simulink model "Full_Model"  (R2024b)
settings: Solver=VariableStepAuto  StartTime=0.0  StopTime=10.0  RelTol=1e-3
libraries: shared6dof x1
settings Model: Creator=bhavy  LastModifiedBy=gtanu

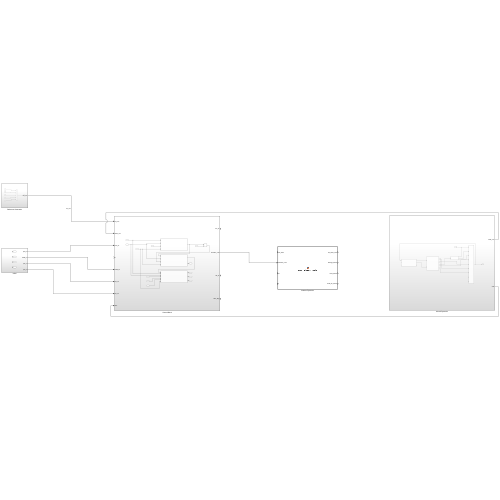
[thumbnail: Simulink's stored preview of the top-level diagram]
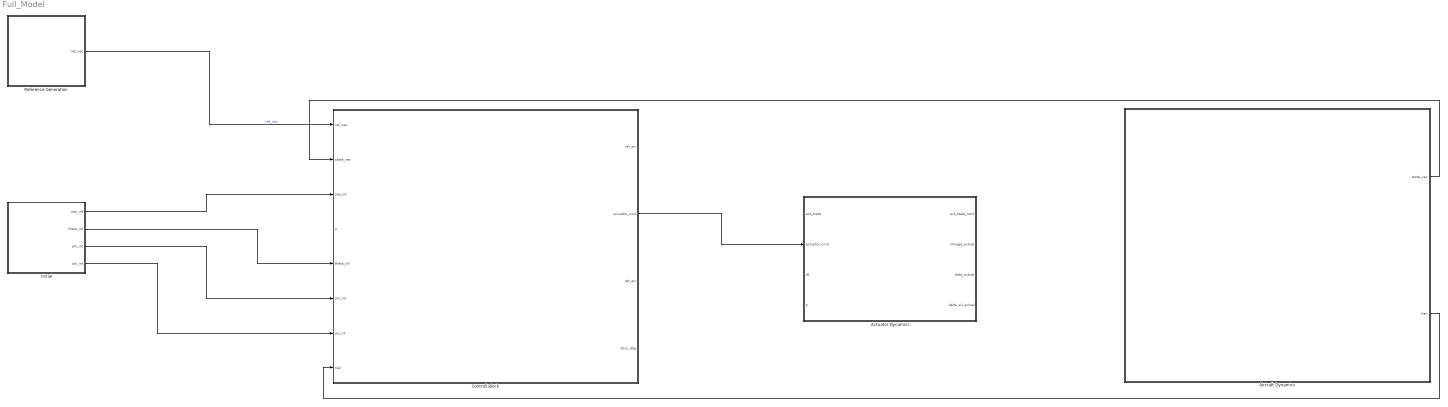
== system Full_Model ==
  Actuator Dynamics : MATLAB Function  TreatAsAtomicUnit=on
  Aircraft Dynamics : Subsystem
  Controll Block : Subsystem
  Initial : Subsystem
  Reference Generation : Subsystem
  wires:
  Reference Generation/1(ref_vec) -> Controll Block/1(ref_vec)  "ref_vec"
  Controll Block/2(actuator_cmd) -> Actuator Dynamics/2(actuator_cmd)
  Aircraft Dynamics/1(state_vec) -> Controll Block/2(state_vec)
  Aircraft Dynamics/2(Vair) -> Controll Block/8(Vair)
  Initial/1(pos_int) -> Controll Block/3(pos_int)
  Initial/2(theta_int) -> Controll Block/5(theta_int)
  Initial/3(phi_int) -> Controll Block/6(phi_int)
  Initial/4(psi_int) -> Controll Block/7(psi_int)

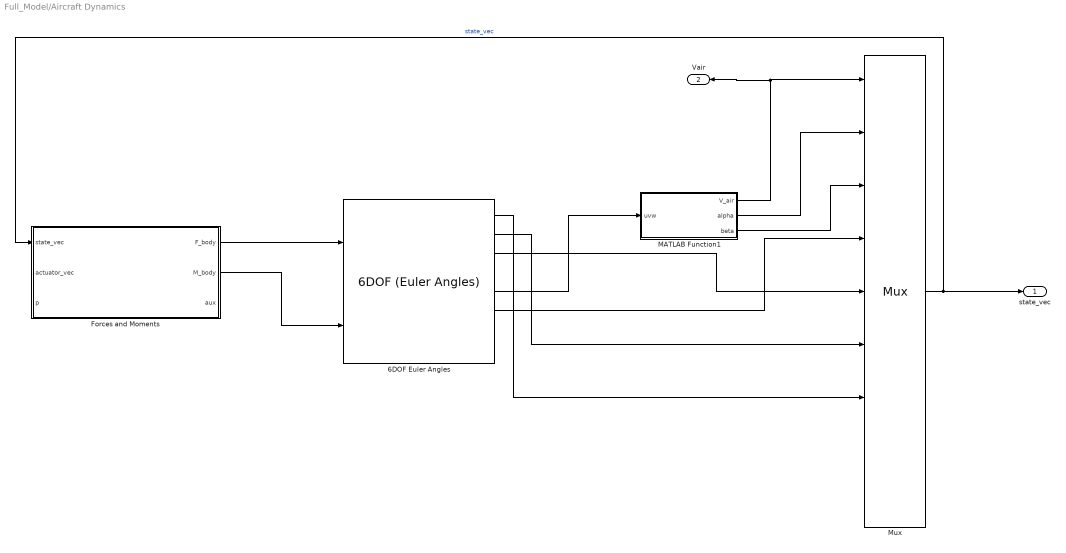
== system Full_Model/Aircraft Dynamics ==
  6DOF Euler Angles : shared6dof/6DOF (Euler Angles)  units=Metric (MKS)  mtype=Fixed  rep=Euler Angles  xme_0=[0 0 0]  Vm_0=[0 0 0]  eul_0=[0 0 0]  pm_0=[0 0 0]  mass_0=1.0  mass_e=0.5  mass_f=2.0  inertia=eye(3)  inertia_e=eye(3)  inertia_f=2*eye(3)  k_quat=1.0  vre_flag=on  abi_flag=off  aMode=0  xme_statename=''  Vm_statename=''  eul_statename=''  quat_statename=''  pm_statename=''  mass_statename=''
  Forces and Moments : MATLAB Function  TreatAsAtomicUnit=on
  MATLAB Function1 : MATLAB Function  TreatAsAtomicUnit=on
  Mux : Mux  Inputs=9
  state_vec : Outport
  Vair : Outport  Port=2
  wires:
  Forces and Moments/1(F_body) -> 6DOF Euler Angles/1
  Forces and Moments/2(M_body) -> 6DOF Euler Angles/2
  6DOF Euler Angles/5 -> MATLAB Function1/1(uvw)
  MATLAB Function1/1(V_air) -> Vair/1, Mux/1
  MATLAB Function1/2(alpha) -> Mux/2
  MATLAB Function1/3(beta) -> Mux/3
  6DOF Euler Angles/6 -> Mux/4
  6DOF Euler Angles/3 -> Mux/5
  6DOF Euler Angles/2 -> Mux/6
  6DOF Euler Angles/1 -> Mux/7
  Mux/1 -> Forces and Moments/1(state_vec), state_vec/1  "state_vec"

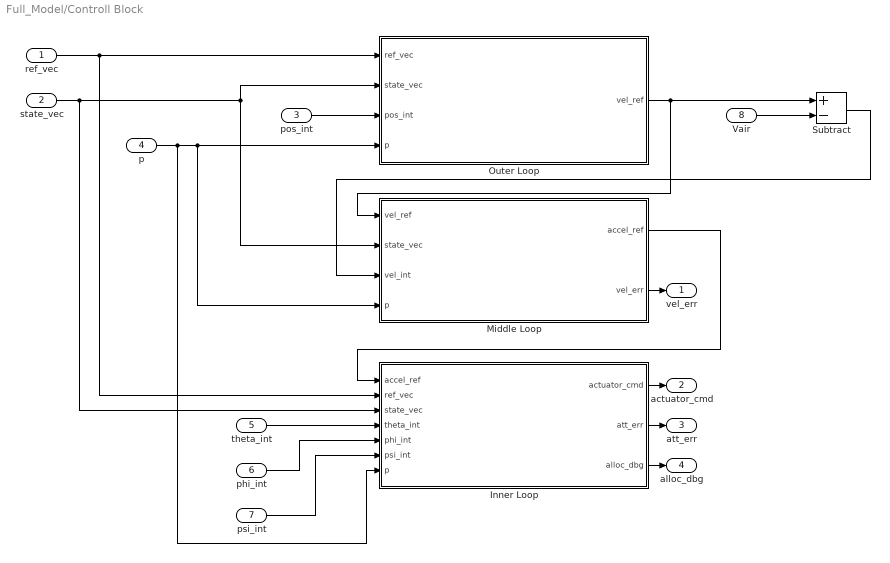
== system Full_Model/Controll Block ==
  ref_vec : Inport
  state_vec : Inport  Port=2
  pos_int : Inport  Port=3
  p : Inport  Port=4
  theta_int : Inport  Port=5
  phi_int : Inport  Port=6
  psi_int : Inport  Port=7
  Vair : Inport  Port=8
  Inner Loop : MATLAB Function  TreatAsAtomicUnit=on
  Middle Loop : MATLAB Function  TreatAsAtomicUnit=on
  Outer Loop : MATLAB Function  TreatAsAtomicUnit=on
  Subtract : Sum  Inputs=+-
  vel_err : Outport
  actuator_cmd : Outport  Port=2
  att_err : Outport  Port=3
  alloc_dbg : Outport  Port=4
  wires:
  p/1 -> Outer Loop/4(p), Middle Loop/4(p), Inner Loop/7(p)
  state_vec/1 -> Inner Loop/3(state_vec), Middle Loop/2(state_vec), Outer Loop/2(state_vec)
  Subtract/1 -> Middle Loop/3(vel_int)
  Middle Loop/2(vel_err) -> vel_err/1
  Outer Loop/1(vel_ref) -> Subtract/1, Middle Loop/1(vel_ref)
  Middle Loop/1(accel_ref) -> Inner Loop/1(accel_ref)
  ref_vec/1 -> Inner Loop/2(ref_vec), Outer Loop/1(ref_vec)
  pos_int/1 -> Outer Loop/3(pos_int)
  Inner Loop/3(alloc_dbg) -> alloc_dbg/1
  theta_int/1 -> Inner Loop/4(theta_int)
  psi_int/1 -> Inner Loop/6(psi_int)
  Inner Loop/2(att_err) -> att_err/1
  Inner Loop/1(actuator_cmd) -> actuator_cmd/1
  phi_int/1 -> Inner Loop/5(phi_int)
  Vair/1 -> Subtract/2

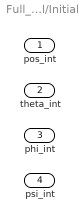
== system Full_Model/Initial ==
  pos_int : Outport
  theta_int : Outport  Port=2
  phi_int : Outport  Port=3
  psi_int : Outport  Port=4

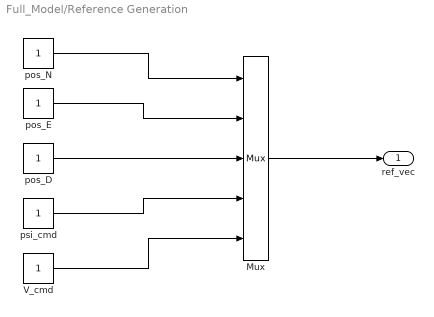
== system Full_Model/Reference Generation ==
  Mux : Mux  Inputs=5
  V_cmd : Constant
  pos_D : Constant
  pos_E : Constant
  pos_N : Constant
  psi_cmd : Constant
  ref_vec : Outport
  wires:
  pos_E/1 -> Mux/2
  V_cmd/1 -> Mux/5
  pos_D/1 -> Mux/3
  pos_N/1 -> Mux/1
  psi_cmd/1 -> Mux/4
  Mux/1 -> ref_vec/1

== matlab function Full_Model/Controll Block/Outer Loop ==
  data: ref_vec input; vel_ref output; state_vec input; pos_int input; p input
function vel_ref = dyulon_outer_loop(ref_vec, state_vec, pos_int, p) %#codegen
%DYULON_OUTER_LOOP  Position controller (outer loop).
%  Converts position error into a velocity reference command.
%  FIXED (from original): p was read via coder.extrinsic('evalin') +
%  evalin('base','p'). coder.extrinsic marks a call as MATLAB-only --
%  Embedded Coder cannot generate standalone C for it, which breaks
%  "hardware ready / code generation" for this whole function. Fixed by
%  passing p as a normal argument, matching dyulon_controller.m and
%  dyulon_actuator_dynamics.m. This requires a matching 4th inport on the
%  Simulink subsystem (see wiring notes at the end of this file / the
%  overall Simulink layout description).
%
%  INPUTS:
%    ref_vec   [5x1]  [pos_N; pos_E; pos_D; psi_cmd; V_cmd]
%    state_vec [23x1] full state vector (see dyulon_init section 19)
%    pos_int   [3x1]  integrated position error from external Discrete
%                     Integrator block (Simulink), NOT computed here.
%                     Anti-windup saturation applied at the Simulink block
%                     level using p.gains.windup_limit_outer.
%    p                parameter struct from dyulon_init.m -- FIXED: now
%                     an explicit argument, was evalin('base',...).
%
%  OUTPUTS:
%    vel_ref   [3x1]  [vN_ref; vE_ref; vD_ref]  m/s  NED frame
%
%  DESIGN NOTES:
%    - Pure PI on position. Ki starts at 0 (see dyulon_init) to avoid
%      windup during transition; raise only if steady-state position error
%      is unacceptable in simulation.
%    - Velocity commands are saturated before output. Saturation limits
%      are defined here as local constants because they are purely a
%      flight-envelope safety bound (not a tuning parameter).
%    - Integral state (pos_int) lives outside this function as a Simulink
%      Discrete Integrator block. This function only reads it.
%
%  REQUIRES (not yet in dyulon_init.m -- see accompanying integration
%  note): p.gains.outer.Kp_xy, .Ki_xy, .Kp_z, .Ki_z
%
%  STATE VECTOR INDEX REFERENCE (from dyulon_init section 19):
%    [10] pos_N  [11] pos_E  [12] pos_D
%    [13] vel_N  [14] vel_E  [15] vel_D

%% --- Unpack reference ---
pos_N_ref = ref_vec(1);
pos_E_ref = ref_vec(2);
pos_D_ref = ref_vec(3);
% ref_vec(4) = psi_cmd  - used by inner loop directly, not here
% ref_vec(5) = V_cmd    - used by inner loop directly, not here

%% --- Unpack state (position) ---
pos_N = state_vec(10);
pos_E = state_vec(11);
pos_D = state_vec(12);

%% --- Position error (NED) ---
err_N = pos_N_ref - pos_N;
err_E = pos_E_ref - pos_E;
err_D = pos_D_ref - pos_D;

%% --- PI control ---
% Integral term (pos_int) fed in from external Simulink Discrete Integrator
vN_ref = p.gains.outer.Kp_xy * err_N + p.gains.outer.Ki_xy * pos_int(1);
vE_ref = p.gains.outer.Kp_xy * err_E + p.gains.outer.Ki_xy * pos_int(2);
vD_ref = p.gains.outer.Kp_z  * err_D + p.gains.outer.Ki_z  * pos_int(3);

%% --- Output saturation ---
% Horizontal: keep well below stall (stall ~20 m/s, cap at 8 m/s for safety)
% Vertical: rate of climb target is 2 m/s from spec; cap descent at 3 m/s
vel_max_xy =  8.0;   % m/s
vel_max_dn =  3.0;   % m/s (positive = descend in NED)
vel_max_up = -2.0;   % m/s (negative = climb in NED)

vN_ref = max(min(vN_ref,  vel_max_xy), -vel_max_xy);
vE_ref = max(min(vE_ref,  vel_max_xy), -vel_max_xy);
vD_ref = max(min(vD_ref,  vel_max_dn),  vel_max_up);

vel_ref = [vN_ref; vE_ref; vD_ref];

end

== matlab function Full_Model/Aircraft Dynamics/Forces and Moments ==
  data: state_vec input; F_body output; actuator_vec input; p input; M_body output; aux output
function [F_body, M_body, aux] = dyulon_forces_moments(state_vec, actuator_vec, p)
%DYULON_FORCES_MOMENTS  Compute total forces and moments on the Dyulon airframe.
%  Rev 4 - rear motors now independently tilt (pusher convention, beta=0=down)
%  FIXED (from original): two bugs found while porting into this function:
%   (1) 'p' was used throughout but never passed in -- this function could
%       not run at all as a standalone Simulink MATLAB Function block
%       (no base-workspace evalin call either, unlike the loop functions).
%       Fixed: p is now an explicit third argument.
%   (2) actuator_vec was documented AND unpacked as 7x1 [Omega x4, beta_FL,
%       beta_FR, delta_ail] -- only front tilt. But the physics loop below
%       (`for i=1:4 ... beta_i = actuators.beta(i)`) needs beta(3) and
%       beta(4) for the rear motors, which were never assigned. Downstream,
%       dyulon_inner_loop already outputs a 9x1 actuator_cmd
%       [Omega x4, beta_FL, beta_FR, beta_RL, beta_RR, delta_ail] -- so the
%       fix is to widen this function's input to match what the rest of
%       the system already produces, not to change the inner loop.
%#codegen
% state_vec:    23x1  (see dyulon_init section 19 for index definitions)
% actuator_vec:  9x1  [Omega_FL, Omega_FR, Omega_RL, Omega_RR,
%                       beta_FL, beta_FR, beta_RL, beta_RR, delta_ail]
%
%  SIGN CONVENTION (kept as originally written, both local zeros):
%    Front motors: beta measured from straight-up    (0=up,   -90=fwd)
%    Rear  motors: beta measured from straight-down  (0=down, -90=fwd)
%    Thrust vector formula is IDENTICAL for both, because each motor's
%    beta is already expressed from its own local zero:
%      T_vec_i = T_i * [-sin(beta_i); 0; -cos(beta_i)]
%    No sign flip or per-motor conditional needed -- this was correct in
%    the original and is unchanged here.
%
%  INPUTS:
%    state_vec(23x1)     full state (dyulon_init.m Sec 19 indices)
%    actuator_vec(9x1)   [Omega_FL; Omega_FR; Omega_RL; Omega_RR;
%                          beta_FL; beta_FR; beta_RL; beta_RR; delta_ail]
%    p                   parameter struct from dyulon_init.m
%
%  OUTPUTS:
%    F_body  [3x1]  total force  in body frame  [Fx; Fy; Fz]  N
%    M_body  [3x1]  total moment in body frame  [Mx; My; Mz]  N.m
%    aux     struct of intermediate quantities for logging/debug

%% --- Unpack only what this function needs from state ---
state.V_air     = state_vec(1);
state.alpha     = state_vec(2);
state.beta_side = state_vec(3);
state.p_rate    = state_vec(4);
state.q_rate    = state_vec(5);
state.r_rate    = state_vec(6);
% [7:15] attitude and position -- not needed by forces_moments
% [16:23] actuator feedback     -- not needed by forces_moments (comes in
%                                   via actuator_vec argument instead)

%% --- Unpack actuators (FIXED: 9 elements, all 4 tilt angles present) ---
actuators.Omega(1)  = actuator_vec(1);   % Omega_FL
actuators.Omega(2)  = actuator_vec(2);   % Omega_FR
actuators.Omega(3)  = actuator_vec(3);   % Omega_RL
actuators.Omega(4)  = actuator_vec(4);   % Omega_RR
actuators.beta(1)   = actuator_vec(5);   % beta_FL
actuators.beta(2)   = actuator_vec(6);   % beta_FR
actuators.beta(3)   = actuator_vec(7);   % beta_RL  -- FIXED: was missing
actuators.beta(4)   = actuator_vec(8);   % beta_RR  -- FIXED: was missing
actuators.delta_ail = actuator_vec(9);   % index shifted 7->9

V      = state.V_air;
alpha  = state.alpha;
beta_s = state.beta_side;
p_rate = state.p_rate;
q_rate = state.q_rate;
r_rate = state.r_rate;

q_bar = 0.5 * p.rho * max(V, 0.1)^2;

%% =========================================================================
%  A. PROPELLER FORCES AND MOMENTS
%% =========================================================================
F_prop = zeros(3,1);
M_prop = zeros(3,1);
M_gyro = zeros(3,1);

V_clamped = min(V, p.prop_V_bp(end));

scale_front = interp1(p.prop_V_bp, p.KpT_front_scale, V_clamped, 'linear');
KpT_front   = p.KpT_front_0 * scale_front;
KpM_front   = p.KpM_front_0 * scale_front;

scale_rear  = interp1(p.prop_V_bp, p.KpT_rear_scale,  V_clamped, 'linear');
KpT_rear    = p.KpT_rear_0  * scale_rear;
KpM_rear    = p.KpM_rear_0  * scale_rear;

% Approximate per-rotor inertia (spinner + blades, kg.m^2)
I_rotor = 1.5e-4;
omega_body = [p_rate; q_rate; r_rate];

for i = 1:4
    Omega_i = actuators.Omega(i);

    if p.motor_type(i) == 1
        KpT_i = KpT_front;  KpM_i = KpM_front;
    else
        KpT_i = KpT_rear;   KpM_i = KpM_rear;
    end

    T_i = KpT_i * Omega_i^2;
    Q_i = KpM_i * Omega_i^2;

    % All motors have independent tilt angle from actuators.beta(i).
    % Front motors: beta measured from straight-up    (0=up,   -90=fwd)
    % Rear  motors: beta measured from straight-down  (0=down, -90=fwd)
    % Formula below is IDENTICAL for both -- convention baked into beta,
    % unchanged from the original (verified correct, kept as-is).
    beta_i = actuators.beta(i);

    T_vec = T_i * [-sin(beta_i); 0; -cos(beta_i)];

    % Reaction torque along thrust axis (opposes spin direction)
    Q_vec = -p.spin_dir(i) * Q_i * [-sin(beta_i); 0; -cos(beta_i)];

    r_i = p.r_motor(i,:)';

    F_prop = F_prop + T_vec;
    M_prop = M_prop + cross(r_i, T_vec) + Q_vec;

    % Gyroscopic coupling: H = I_rotor * Omega * spin_axis
    spin_axis = [-sin(beta_i); 0; -cos(beta_i)];
    H_rotor   = p.spin_dir(i) * I_rotor * Omega_i * spin_axis;
    M_gyro    = M_gyro + cross(omega_body, H_rotor);
end

%% =========================================================================
%  B. WING AERODYNAMICS
%% =========================================================================
if V > 2.0
    alpha_deg     = rad2deg(alpha);
    alpha_clamped = max(p.aero_alpha_deg(1), min(p.aero_alpha_deg(end), alpha_deg));

    CL = interp1(p.aero_alpha_deg, p.aero_CL, alpha_clamped, 'linear');
    CD = interp1(p.aero_alpha_deg, p.aero_CD, alpha_clamped, 'linear');
    Cm = interp1(p.aero_alpha_deg, p.aero_Cm, alpha_clamped, 'linear');

    Lift = q_bar * p.S * CL;
    Drag = q_bar * p.S * CD;

    Fx_aero =  Lift * sin(alpha) - Drag * cos(alpha);
    Fz_aero = -Lift * cos(alpha) - Drag * sin(alpha);
    Fy_aero =  q_bar * p.S * (-0.15) * beta_s;

    F_aero = [Fx_aero; Fy_aero; Fz_aero];

    Cm_total = Cm + p.Cm_q * (q_rate * p.cbar / (2 * max(V, 0.1)));
    My_aero  = q_bar * p.S * p.cbar * Cm_total;

    Cl_total = p.Cl_b  * beta_s ...
             + p.Cl_p  * (p_rate * p.b / (2 * max(V, 0.1))) ...
             + p.Cl_da * actuators.delta_ail;
    Mx_aero  = q_bar * p.S * p.b * Cl_total;

    Cn_total = p.Cn_b * beta_s + p.Cn_r * (r_rate * p.b / (2 * max(V, 0.1)));
    Mz_aero  = q_bar * p.S * p.b * Cn_total;

    M_aero = [Mx_aero; My_aero; Mz_aero];
else
    F_aero = zeros(3,1);  M_aero = zeros(3,1);
    CL = 0; CD = 0; Cm = 0; Lift = 0; Drag = 0;
end

%% =========================================================================
%  C. TOTAL FORCES AND MOMENTS
%  Gravity handled by Aerospace Blockset 6DOF (Euler Angles) block
%  internally in NED frame. Do NOT add gravity here.
%% =========================================================================
F_body = F_prop + F_aero;
M_body = M_prop + M_aero + M_gyro;

%% =========================================================================
%  D. AUX STRUCT (for Simulink logging and To Workspace blocks)
%% =========================================================================
aux.F_prop    = F_prop;
aux.F_aero    = F_aero;
aux.M_prop    = M_prop;
aux.M_aero    = M_aero;
aux.M_gyro    = M_gyro;
aux.KpT_front = KpT_front;
aux.KpT_rear  = KpT_rear;
aux.q_bar     = q_bar;
aux.CL        = CL;
aux.CD        = CD;
aux.Lift      = Lift;
aux.Drag      = Drag;

end

== matlab function Full_Model/Controll Block/Middle Loop ==
  data: vel_ref input; accel_ref output; state_vec input; vel_int input; p input; vel_err output
function [accel_ref, vel_err] = dyulon_mid_loop(vel_ref, state_vec, vel_int, p) %#codegen
%DYULON_MID_LOOP  Velocity controller (mid loop).
%  Converts velocity error into an acceleration reference command.
%  FIXED (from original): p was read via coder.extrinsic('evalin') +
%  evalin('base','p'), which blocks C code generation for this function.
%  Fixed by passing p as a normal argument (see dyulon_outer_loop_FIXED.m
%  for the same fix and the reasoning). Requires a matching 4th inport on
%  the Simulink subsystem.
%
%  INPUTS:
%    vel_ref   [3x1]  [vN_ref; vE_ref; vD_ref]   from outer loop   m/s
%    state_vec [23x1] full state vector (see dyulon_init section 19)
%    vel_int   [3x1]  integrated velocity error from external Simulink
%                     Discrete Integrator block.
%                     Anti-windup saturation: +/-p.gains.windup_limit_mid
%                     applied at the Simulink block level.
%    p                parameter struct from dyulon_init.m -- FIXED: now
%                     an explicit argument, was evalin('base',...).
%
%  OUTPUTS:
%    accel_ref [3x1]  [aN_ref; aE_ref; aD_ref]   NED frame  m/s^2
%                     These are TOTAL desired accelerations including gravity
%                     compensation - the inner loop converts to motor forces.
%    vel_err   [3x1]  current velocity error (fed to Simulink integrator
%                     input so this function and the integrator block stay
%                     in sync without recomputing the error externally)
%
%  DESIGN NOTES:
%    - NED convention: positive aD_ref = downward acceleration.
%      To hold altitude, aD_ref = 0 (gravity handled by 6DOF block).
%      To climb (pos_D decreasing = going up), aD_ref < 0.
%    - accel_ref is clamped to physically reachable values. Horizontal
%      acceleration limit chosen to keep bank angles below ~30 deg
%      (tan(30) * g ~= 5.7 m/s^2). Vertical limit from T/W ratio.
%    - This function only outputs the proportional + integral correction.
%      The inner loop handles gravity compensation internally via the
%      collective thrust term.
%
%  REQUIRES (not yet in dyulon_init.m -- see accompanying integration
%  note): p.gains.mid.Kp_xy, .Ki_xy, .Kp_z, .Ki_z
%
%  STATE VECTOR INDEX REFERENCE:
%    [13] vel_N  [14] vel_E  [15] vel_D  m/s NED

%% --- Unpack velocity from state ---
vel_N = state_vec(13);
vel_E = state_vec(14);
vel_D = state_vec(15);

%% --- Velocity error ---
err_N = vel_ref(1) - vel_N;
err_E = vel_ref(2) - vel_E;
err_D = vel_ref(3) - vel_D;

vel_err = [err_N; err_E; err_D];

%% --- PI acceleration command ---
aN_ref = p.gains.mid.Kp_xy * err_N + p.gains.mid.Ki_xy * vel_int(1);
aE_ref = p.gains.mid.Kp_xy * err_E + p.gains.mid.Ki_xy * vel_int(2);
aD_ref = p.gains.mid.Kp_z  * err_D + p.gains.mid.Ki_z  * vel_int(3);

%% --- Output saturation ---
% Horizontal: bank angle limited to ~30 deg implicitly (5.7 m/s^2)
% Vertical: T/W = 1.4 gives max upward accel of 0.4*g ~= 3.9 m/s^2 net of gravity
accel_max_xy  =  5.7;          % m/s^2
accel_max_dn  =  0.4 * p.g;    % m/s^2  (positive = push downward in NED, rare)
accel_max_up  = -0.4 * p.g;    % m/s^2  (negative = push upward in NED, climb)

aN_ref = max(min(aN_ref,  accel_max_xy), -accel_max_xy);
aE_ref = max(min(aE_ref,  accel_max_xy), -accel_max_xy);
aD_ref = max(min(aD_ref,  accel_max_dn),  accel_max_up);

accel_ref = [aN_ref; aE_ref; aD_ref];

end

== matlab function Full_Model/Controll Block/Inner Loop ==
  data: accel_ref input; actuator_cmd output; ref_vec input; state_vec input; theta_int input; phi_int input; psi_int input; p input; att_err output; alloc_dbg output
function [actuator_cmd, att_err, alloc_dbg] = dyulon_inner_loop(...
    accel_ref, ref_vec, state_vec, theta_int, phi_int, psi_int, p) %#codegen
%DYULON_INNER_LOOP  Attitude + control allocation (inner loop).
%
%  Takes desired acceleration from the mid loop and the full state, and
%  outputs motor speed (Omega) and tilt angle (beta) commands for all 4
%  motors plus aileron deflection.
%
%  The function is structured in five sequential stages:
%    1. Unpack state and compute blend factor
%    2. Compute attitude reference (theta_ref, phi_ref, psi_ref)
%    3. AoA protection - saturate theta_ref if stall risk detected,
%       flag that motor speed compensation is needed
%    4. PID attitude control -> desired angular accelerations
%    5. Control allocation:
%         a. Compute collective thrust needed (vertical + forward)
%         b. Distribute among motors using 2-DOF per motor (Omega + beta)
%            DOF weighting from p.alloc_weights (currently 50/50)
%            Tilt perturbation bounded by stage-dependent limits from
%            p.tilt_limits, interpolated continuously via blend
%         c. Apply motor speed compensation if AoA was saturated
%         d. Saturate all outputs against hard mechanical/electrical limits
%
%  INPUTS:
%    accel_ref  [3x1]  [aN; aE; aD]  NED  m/s²   from mid loop
%    ref_vec    [5x1]  [pos_N; pos_E; pos_D; psi_cmd; V_cmd]
%    state_vec  [23x1] full state (see dyulon_init section 19)
%    theta_int  [1x1]  integrated pitch error  (external Discrete Integrator)
%    phi_int    [1x1]  integrated roll error   (external Discrete Integrator)
%    psi_int    [1x1]  integrated yaw error    (external Discrete Integrator)
%
%  OUTPUTS:
%    actuator_cmd [9x1]  [Omega_FL; Omega_FR; Omega_RL; Omega_RR;
%                          beta_FL;  beta_FR;  beta_RL;  beta_RR;
%                          delta_ail]
%    att_err      [3x1]  [theta_err; phi_err; psi_err]  for integrator input
%    alloc_dbg    [6x1]  debug: [blend; theta_ref; phi_ref;
%                                aoa_saturated; Fz_motors; Fx_motors]
%
%  STATE VECTOR INDEX REFERENCE (dyulon_init section 19):
%    [1]  V_air   [2]  alpha   [3]  beta_side
%    [4]  p_rate  [5]  q_rate  [6]  r_rate
%    [7]  phi     [8]  theta   [9]  psi
%    [10:12] pos  [13:15] vel
%    [16] beta_FL [17] beta_FR [18] beta_RL [19] beta_RR
%    [20] Omega_FL [21] Omega_FR [22] Omega_RL [23] Omega_RR
%
%  FIXED (from original): p was read via coder.extrinsic('evalin') +
%  evalin('base','p'), which blocks Embedded Coder C generation for this
%  function -- same issue and same fix as dyulon_outer_loop / dyulon_mid_loop.
%  p is now the 7th argument. Requires a matching 7th inport on the
%  Simulink subsystem.

%% =========================================================================
%  STAGE 1 - UNPACK STATE
%% =========================================================================
V_air   = state_vec(1);
alpha   = state_vec(2);   % rad, angle of attack
p_rate  = state_vec(4);   % rad/s, roll rate
q_rate  = state_vec(5);   % rad/s, pitch rate
r_rate  = state_vec(6);   % rad/s, yaw rate
phi     = state_vec(7);   % rad, roll angle
theta   = state_vec(8);   % rad, pitch angle
psi     = state_vec(9);   % rad, yaw angle

% Current actual tilt and speed (feedback from actuator model output)
beta_actual  = state_vec(16:19);   % [FL; FR; RL; RR] rad
% Omega_actual = state_vec(20:23); % available if needed for feedforward

psi_cmd = ref_vec(4);

%% =========================================================================
%  STAGE 2 - BLEND FACTOR (single source of truth, same formula as doc)
%% =========================================================================
blend = max(0.0, min(1.0, (V_air - p.V_blend_lo) / (p.V_blend_hi - p.V_blend_lo)));

%% =========================================================================
%  STAGE 3 - ATTITUDE REFERENCE
%
%  theta_ref: interpolate between hover (0 rad) and cruise (alpha_bestLD)
%  phi_ref:   derived from lateral acceleration demand (coordinated turn)
%  psi_ref:   commanded heading from ref_vec
%
%  NOTE: accel_ref is in NED. To get body-frame lateral accel demand
%  (used for bank angle reference), we rotate using current heading psi.
%% =========================================================================

% Pitch reference - blend from hover to best-L/D AoA in cruise
theta_hover  = 0.0;
theta_cruise = deg2rad(p.alpha_bestLD_deg);   % trim at best L/D
theta_ref    = (1.0 - blend) * theta_hover + blend * theta_cruise;

% Roll reference from lateral acceleration demand (NED -> body lateral)
% Body-frame lateral accel ≈ -sin(psi)*aN + cos(psi)*aE  for small phi
ay_body  = -sin(psi) * accel_ref(1) + cos(psi) * accel_ref(2);
phi_ref  = atan2(ay_body, p.g);   % coordinated turn bank angle
phi_ref  = max(min(phi_ref, deg2rad(30)), deg2rad(-30));  % limit bank to ±30 deg

psi_ref  = psi_cmd;

%% =========================================================================
%  STAGE 4 - AoA PROTECTION
%
%  If current alpha approaches stall, override theta_ref with the
%  protection ceiling and flag that extra motor speed is needed to meet
%  the original lift demand. The motor compensation is applied in Stage 6.
%
%  Protection band from dyulon_init:
%    p.alpha_protect_lo_deg  - lower bound (avoid negative stall)
%    p.alpha_protect_hi_deg  - upper bound (stall margin = stall_AoA - 2 deg)
%% =========================================================================
alpha_deg       = rad2deg(alpha);
aoa_saturated   = 0.0;   % flag: 0 = normal, 1 = upper, -1 = lower

if alpha_deg >= p.alpha_protect_hi_deg
    % Approaching stall - cap theta_ref so AoA stops increasing
    % We cannot pitch further nose-up, but we CAN increase motor speed
    theta_ref     = deg2rad(p.alpha_protect_hi_deg);
    aoa_saturated = 1.0;
elseif alpha_deg <= p.alpha_protect_lo_deg
    % Approaching negative stall (e.g. aggressive pushover)
    theta_ref     = deg2rad(p.alpha_protect_lo_deg);
    aoa_saturated = -1.0;
end

%% =========================================================================
%  STAGE 5 - PID ATTITUDE CONTROL
%
%  Uses direct rate feedback for derivative term (not d(error)/dt) to
%  avoid differentiating noisy angle measurements. This structure is
%  directly portable to ArduPilot's rate-feedback PID architecture.
%
%    pitch output = Kp*(theta_ref-theta) + Ki*theta_int - Kd*q_rate
%    roll  output = Kp*(phi_ref-phi)     + Ki*phi_int   - Kd*p_rate
%    yaw   output = Kp*(psi_ref-psi)     + Ki*psi_int   - Kd*r_rate
%
%  Output is a desired angular acceleration [rad/s²] for pitch and roll,
%  and a desired yaw rate correction [rad/s] for yaw (Kd_psi = 0 default).
%  These drive the force allocation in Stage 6.
%% =========================================================================

% Attitude errors (fed back out as att_err for Simulink integrator inputs)
theta_err = theta_ref - theta;
phi_err   = phi_ref   - phi;
psi_err   = psi_ref   - psi;

% Wrap yaw error to [-pi, pi]
psi_err = mod(psi_err + pi, 2*pi) - pi;

att_err = [theta_err; phi_err; psi_err];

% PID outputs (desired angular accelerations / rate corrections)
pitch_cmd = p.gains.inner.Kp_theta * theta_err ...
          + p.gains.inner.Ki_theta  * theta_int ...
          - p.gains.inner.Kd_theta  * q_rate;

roll_cmd  = p.gains.inner.Kp_phi   * phi_err ...
          + p.gains.inner.Ki_phi    * phi_int ...
          - p.gains.inner.Kd_phi    * p_rate;

yaw_cmd   = p.gains.inner.Kp_psi   * psi_err ...
          + p.gains.inner.Ki_psi    * psi_int ...
          - p.gains.inner.Kd_psi    * r_rate;

% Convert angular acceleration demands to differential force demands
% pitch_force = Iyy * pitch_cmd / moment_arm (front-rear x distance)
x_arm   = p.x_front - p.x_rear;   % m  total front-to-rear moment arm
y_arm_f = abs(p.r_motor(1,2));     % m  front lateral arm (roll)
y_arm_r = abs(p.r_motor(3,2));     % m  rear  lateral arm (roll)
y_arm   = 0.5 * (y_arm_f + y_arm_r);  % average for roll allocation

delta_F_pitch = p.Iyy * pitch_cmd / x_arm;   % N  differential vertical force front vs rear
delta_F_roll  = p.Ixx * roll_cmd  / y_arm;   % N  differential vertical force left vs right
delta_F_yaw   = p.Izz * yaw_cmd;             % N·m  yaw torque demand (met by reaction torques)

%% =========================================================================
%  STAGE 6 - COLLECTIVE THRUST DEMAND
%
%  Vertical force needed from motors:
%    In hover:  motors provide all lift = mass * (g + az_cmd)
%    In cruise: wing provides blend fraction of lift, motors provide rest
%
%  Forward force needed from motors:
%    In hover:  from aN/aE demands (small, met by tilt)
%    In cruise: from drag balance (met primarily by rear motors)
%
%  accel_ref is NED (positive D = downward). To get vertical demand in
%  body frame (z-down), Fz_needed is the upward force = mass*(g - aD_NED)
%  because aD_NED > 0 means accelerating downward (reducing lift demand).
%
%  Wing lift available at current alpha and airspeed:
%    Lift_avail = 0.5*rho*V^2*S*CL(alpha) - looked up from LUT
%  Motor vertical demand = total_needed - blend*Lift_avail
%% =========================================================================

% Total upward force needed [body frame, positive = up, so subtract aD]
Fz_total_needed = p.mass * (p.g - accel_ref(3));   % accel_ref(3) = aD_NED

% Wing lift available now (interpolate from LUT at current alpha)
alpha_deg_clamped = max(p.aero_alpha_deg(1), min(p.aero_alpha_deg(end), alpha_deg));
CL_now     = interp1(p.aero_alpha_deg, p.aero_CL, alpha_deg_clamped, 'linear');
Lift_avail = 0.5 * p.rho * max(V_air, 0.1)^2 * p.S * CL_now;

% Motor vertical demand (wing takes blend fraction, motors take the rest)
Fz_motors = Fz_total_needed - blend * Lift_avail;
Fz_motors = max(Fz_motors, 0.0);   % motors cannot pull downward

% Forward force demand (body x-axis)
% In NED: ax_body ≈ cos(psi)*aN + sin(psi)*aE  for small phi/theta
ax_body   = cos(psi) * accel_ref(1) + sin(psi) * accel_ref(2);
% Drag at current condition (for feedforward in cruise)
CD_now    = interp1(p.aero_alpha_deg, p.aero_CD, alpha_deg_clamped, 'linear');
Drag_now  = 0.5 * p.rho * max(V_air, 0.1)^2 * p.S * CD_now;
Fx_motors = p.mass * ax_body + Drag_now;   % overcome drag + accelerate forward

% Front/rear collective split (from frac_front / frac_rear)
Fz_front = p.frac_front * Fz_motors;
Fz_rear  = p.frac_rear  * Fz_motors;
Fx_front = p.frac_front * Fx_motors;
Fx_rear  = p.frac_rear  * Fx_motors;

%% =========================================================================
%  STAGE 7 - 2-DOF CONTROL ALLOCATION PER MOTOR GROUP
%
%  Each motor has two DOFs: Omega (speed -> thrust magnitude) and beta
%  (tilt -> thrust direction). For a given thrust VECTOR demand [Fx; Fz],
%  there are infinitely many (Omega, beta) combinations that satisfy it.
%  The allocation weight (p.alloc_weights) splits the correction between
%  the two DOFs: at 0.5/0.5, half the correction is attempted via beta
%  change and half via Omega change.
%
%  PRIMARY tilt target (blend-driven, stage-level command):
%    Front: beta_front_primary = beta_front_rest + (-pi/2 - beta_front_rest)*blend
%           = 0 + (-90 - 0)*blend = -90*blend deg
%           (0 deg in hover = straight up, -90 deg in cruise = forward)
%
%    Rear:  beta_rear_primary  = beta_rear_rest + (-pi/2 - beta_rear_rest)*blend
%           = -20 + (-90 - (-20))*blend = -20 - 70*blend  [deg]
%           At blend=0 (hover):      beta = -20 deg  (94% up, 34% fwd)
%           At blend=0.5 (transit):  beta = -55 deg  (82% fwd, 57% up)
%           At blend=1 (cruise):     beta = -90 deg  (100% fwd, 0% up)
%           The -100 deg hard stop gives ±10 deg perturbation room in cruise.
%
%  PERTURBATION on top of primary (for attitude correction via tilt):
%    Interpolated from p.tilt_limits vs blend continuously.
%    Front perturb: 2 deg (hover) -> 10 deg (cruise)
%    Rear  perturb: 8 deg (hover) ->  2 deg (cruise)
%
%  MOTOR SPEED from the remaining force demand not met by tilt change.
%
%  All outputs clamped to hard limits from p before exit.
%% =========================================================================

% --- Tilt perturbation limits at current blend (continuous interp) ---
front_perturb_rad = interp1(p.tilt_limits.V_bp, ...
                            p.tilt_limits.front_perturb_rad_bp, ...
                            V_air, 'linear', 'extrap');
front_perturb_rad = max(0, min(front_perturb_rad, deg2rad(15)));

rear_perturb_rad  = interp1(p.tilt_limits.V_bp, ...
                             p.tilt_limits.rear_perturb_rad_bp, ...
                             V_air, 'linear', 'extrap');
rear_perturb_rad  = max(0, min(rear_perturb_rad, deg2rad(15)));

% --- Primary tilt commands (stage-level blend schedule) ---
% Front: 0 (hover) -> -pi/2 (cruise), referenced from front zero (up)
beta_front_primary = p.beta_front_rest + (-pi/2 - p.beta_front_rest) * blend;

% Rear: -100deg (hover) -> -90deg (cruise), referenced from rear zero (down)
beta_rear_primary  = p.beta_rear_rest  + (-pi/2 - p.beta_rear_rest)  * blend;

% --- Attitude correction via tilt (pitch) ---
% Positive pitch_correction: want more nose-up = front motors tilt back
% (less forward component = increase beta toward 0) or rear motors
% tilt more forward (decrease beta, more negative for rear convention).
% Scale delta_F_pitch to a tilt perturbation angle via a linearisation:
% dFz/dbeta ≈ -T_front * cos(beta_primary) at operating point
% Use a soft gain rather than exact inversion (plant uncertainty too high
% for exact inversion at this stage)
pitch_tilt_gain_front = 0.003;  % rad/N  - tune in sim
pitch_tilt_gain_rear  = 0.003;  % rad/N

delta_beta_pitch_front = p.alloc_weights.tilt_share * pitch_tilt_gain_front * delta_F_pitch;
delta_beta_pitch_rear  = p.alloc_weights.tilt_share * pitch_tilt_gain_rear  * (-delta_F_pitch);

% Clamp tilt perturbation to stage-dependent limit
delta_beta_pitch_front = max(min(delta_beta_pitch_front,  front_perturb_rad), -front_perturb_rad);
delta_beta_pitch_rear  = max(min(delta_beta_pitch_rear,   rear_perturb_rad),  -rear_perturb_rad);

% --- Roll correction: only via motor SPEED (L/R differential Omega) ---
% Tilt does not help with roll (both L and R motors on same fore-aft axis).
% Roll entirely via Omega differential, ignoring alloc_weights for roll axis.
% (alloc_weights applies only to pitch/thrust axes where tilt can help)

% --- Compute required thrust magnitudes per motor ---
% Remaining vertical force after tilt perturbation (Omega carries the rest)
% Front motors: each provides Fz_front/2 ± roll differential
KpT_front_now = p.KpT_front_0 * interp1(p.prop_V_bp, p.KpT_front_scale, ...
                min(V_air, p.prop_V_bp(end)), 'linear');
KpT_rear_now  = p.KpT_rear_0  * interp1(p.prop_V_bp, p.KpT_rear_scale, ...
                min(V_air, p.prop_V_bp(end)), 'linear');

% Collective Omega from vertical + forward demand
% |T_front| = sqrt(Fz_front^2 + Fx_front^2) per motor (vector magnitude)
T_front_mag = sqrt((Fz_front/2)^2 + (Fx_front/2)^2);
T_rear_mag  = sqrt((Fz_rear/2)^2  + (Fx_rear/2)^2);

% Omega_collective = sqrt(T_mag / KpT)  only for the Omega share
T_front_omega_share = T_front_mag * p.alloc_weights.omega_share;
T_rear_omega_share  = T_rear_mag  * p.alloc_weights.omega_share;

% Add back the tilt share (tilt handles the rest; Omega only sees its share)
% In practice the full T is still needed, but the tilt adjusts direction
% so the effective Omega demand is based on vector magnitude not just vertical
Omega_front_col = sqrt(max(T_front_mag / max(KpT_front_now, 1e-9), 0));
Omega_rear_col  = sqrt(max(T_rear_mag  / max(KpT_rear_now,  1e-9), 0));

% --- Signed-sqrt for attitude differential Omega corrections ---
% Uses sign(x)*sqrt(|x|) to allow bidirectional corrections without
% clipping negative demands to zero (Rev 3 bugfix carried forward).
signed_sqrt = @(x) sign(x) * sqrt(abs(x));

% Pitch correction via motor speed (Omega share of delta_F_pitch)
dF_pitch_omega_front = p.alloc_weights.omega_share * ( delta_F_pitch / 2);
dF_pitch_omega_rear  = p.alloc_weights.omega_share * (-delta_F_pitch / 2);
dOmega_pitch_front   = signed_sqrt(dF_pitch_omega_front / max(KpT_front_now, 1e-9));
dOmega_pitch_rear    = signed_sqrt(dF_pitch_omega_rear  / max(KpT_rear_now,  1e-9));

% Roll correction fully via motor speed differential
dF_roll  = delta_F_roll / 2;   % per motor, symmetric
dOmega_roll_f = signed_sqrt(dF_roll / max(KpT_front_now, 1e-9));
dOmega_roll_r = signed_sqrt(dF_roll / max(KpT_rear_now,  1e-9));

% --- Yaw correction via differential reaction torque ---
% Yaw authority is weak (no fin). Differential Omega changes reaction torque.
% KpM/KpT ratio gives torque per unit thrust, so:
% delta_Q_yaw must equal delta_F_yaw
% delta_Q = KpM * delta_Omega^2 (approximately: 2*KpM*Omega*dOmega for small dOmega)
% Use simple proportional split: increase CCW pair, decrease CW pair
% Spin dirs: FL=-1(CCW), FR=+1(CW), RL=+1(CW), RR=-1(CCW)
KpM_front_now = p.KpM_front_0 * interp1(p.prop_V_bp, p.KpM_front_scale, ...
                min(V_air, p.prop_V_bp(end)), 'linear');
yaw_gain = 0.001;  % rad/s per N·m yaw demand - soft gain, tune in sim
dOmega_yaw = yaw_gain * yaw_cmd;  % same magnitude, sign varies by spin direction below

% --- Final per-motor tilt angles ---
beta_FL = beta_front_primary + delta_beta_pitch_front;
beta_FR = beta_front_primary + delta_beta_pitch_front;  % same pitch correction
beta_RL = beta_rear_primary  + delta_beta_pitch_rear;
beta_RR = beta_rear_primary  + delta_beta_pitch_rear;

% Hard clamp to mechanical stops (from p.beta_motor_min / max)
beta_FL = max(min(beta_FL, p.beta_motor_max(1)), p.beta_motor_min(1));
beta_FR = max(min(beta_FR, p.beta_motor_max(2)), p.beta_motor_min(2));
beta_RL = max(min(beta_RL, p.beta_motor_max(3)), p.beta_motor_min(3));
beta_RR = max(min(beta_RR, p.beta_motor_max(4)), p.beta_motor_min(4));

% --- Final per-motor Omega ---
% Spin dirs: FL=-1, FR=+1, RL=+1, RR=-1
% Roll: right motors (FR, RR) go up = increase Omega_R to roll left
%   -> FL decreases, FR increases, RL decreases, RR increases (or signs flip)
%   Convention: positive roll_cmd = roll right = right wing goes down
%               = left motors increase, right motors decrease
Omega_FL = Omega_front_col + dOmega_pitch_front - dOmega_roll_f - p.spin_dir(1)*dOmega_yaw;
Omega_FR = Omega_front_col + dOmega_pitch_front + dOmega_roll_f - p.spin_dir(2)*dOmega_yaw;
Omega_RL = Omega_rear_col  + dOmega_pitch_rear  - dOmega_roll_r - p.spin_dir(3)*dOmega_yaw;
Omega_RR = Omega_rear_col  + dOmega_pitch_rear  + dOmega_roll_r - p.spin_dir(4)*dOmega_yaw;

%% =========================================================================
%  STAGE 8 - AoA SATURATION MOTOR SPEED COMPENSATION
%
%  If AoA was saturated (aoa_saturated != 0), the original lift demand
%  cannot be met by pitching further. Instead, distribute the unmet lift
%  demand as additional collective motor speed across all 4 motors, split
%  proportionally by p.alloc_weights.omega_share vs wing contribution.
%
%  Weight: 50% front, 50% rear (p.alloc_weights is 50/50 globally).
%% =========================================================================
if abs(aoa_saturated) > 0.5
    % Estimate unmet lift: how much MORE vertical force is needed above
    % what the current theta_ref + current alpha provides?
    % Approximation: unmet = original Fz_total_needed - current Lift_avail - Fz_motors
    % In practice the integrators will handle slow residual; this compensation
    % is for fast transient saturation events only.
    Lift_at_protected_aoa = 0.5 * p.rho * max(V_air,0.1)^2 * p.S * CL_now;
    Fz_unmet = max(Fz_total_needed - Lift_at_protected_aoa - Fz_motors, 0);

    % Split unmet force across all 4 motors proportionally
    dF_comp_front = Fz_unmet * p.alloc_weights.omega_share * p.frac_front / 2;
    dF_comp_rear  = Fz_unmet * p.alloc_weights.omega_share * p.frac_rear  / 2;

    dOmega_comp_front = signed_sqrt(dF_comp_front / max(KpT_front_now, 1e-9));
    dOmega_comp_rear  = signed_sqrt(dF_comp_rear  / max(KpT_rear_now,  1e-9));

    Omega_FL = Omega_FL + dOmega_comp_front;
    Omega_FR = Omega_FR + dOmega_comp_front;
    Omega_RL = Omega_RL + dOmega_comp_rear;
    Omega_RR = Omega_RR + dOmega_comp_rear;
end

%% =========================================================================
%  STAGE 9 - AILERON (blend-weighted, suppressed in hover)
%
%  In hover (blend=0): ailerons too slow to be effective, command = 0.
%  In cruise (blend=1): ailerons are primary roll actuator.
%  roll_cmd is in rad/s² (desired roll acceleration). Scale to aileron
%  deflection via static effectiveness (p.Cl_da, wing geometry).
%  Aileron effectiveness: M_roll = q_bar * S * b * Cl_da * delta_ail
%    -> delta_ail = Ixx * roll_cmd / (q_bar * S * b * Cl_da)
%  Suppressed in low-q (slow flight) by blend weight.
%% =========================================================================
q_bar_now   = 0.5 * p.rho * max(V_air, 0.1)^2;
ail_denom   = q_bar_now * p.S * p.b * p.Cl_da;
if abs(ail_denom) > 1e-6
    delta_ail_raw = blend * (p.Ixx * roll_cmd / ail_denom);
else
    delta_ail_raw = 0;
end
delta_ail = max(min(delta_ail_raw, p.aileron_max), p.aileron_min);

%% =========================================================================
%  STAGE 10 - FINAL SATURATION OF MOTOR SPEEDS
%% =========================================================================
Omega_FL = max(min(Omega_FL, p.Omega_max(1)), p.Omega_min(1));
Omega_FR = max(min(Omega_FR, p.Omega_max(2)), p.Omega_min(2));
Omega_RL = max(min(Omega_RL, p.Omega_max(3)), p.Omega_min(3));
Omega_RR = max(min(Omega_RR, p.Omega_max(4)), p.Omega_min(4));

%% =========================================================================
%  OUTPUTS
%% =========================================================================
actuator_cmd = [Omega_FL; Omega_FR; Omega_RL; Omega_RR;
                beta_FL;  beta_FR;  beta_RL;  beta_RR;
                delta_ail];

% Debug vector for Simulink logging (To Workspace block)
alloc_dbg = [blend; theta_ref; phi_ref; aoa_saturated; Fz_motors; Fx_motors];

== matlab function Full_Model/Actuator Dynamics ==
  data: act_state input; act_state_next output; actuator_cmd input; dt input; p input; Omega_actual output; beta_actual output; delta_ail_actual output
function [act_state_next, Omega_actual, beta_actual, delta_ail_actual] = ...
    dyulon_actuator_dynamics(act_state, actuator_cmd, dt, p) %#codegen
%DYULON_ACTUATOR_DYNAMICS  Discrete-time actuator lag/rate-limit/saturation.
%  Models the REAL hardware: 4x ESC+motor (speed loop), 4x direct-drive
%  gearmotor tilt actuator (NOT a servo), and the aileron servo.
%
%  COMPATIBILITY CHANGE (this revision): earlier version assumed a single
%  unified beta convention (0=horizontal, pi/2=vertical, shared front/rear
%  limits). The controller cascade (dyulon_inner_loop etc.) instead uses
%  TWO local zeros -- front: 0=up,-90deg=fwd; rear: 0=down,-90deg=fwd --
%  per motor, with PER-MOTOR limits (p.beta_motor_min/max, 4x1 each),
%  not shared front/rear bounds. This function's 2nd-order tilt dynamics
%  are convention-agnostic (they only act on the numeric difference
%  beta_cmd - beta, regardless of what zero means physically), so ONLY
%  the saturation limits changed -- from p.beta_min_front/rear (2 shared
%  values) to p.beta_motor_min/max (4x1, one per motor). No other logic
%  needed to change.
%
%  INPUT SHAPE CHANGE: now takes the actual 9x1 actuator_cmd vector
%  dyulon_inner_loop already produces
%  ([Omega_FL;Omega_FR;Omega_RL;Omega_RR; beta_FL;beta_FR;beta_RL;beta_RR;
%  delta_ail]) directly, instead of two separate 4x1 arguments -- avoids
%  an extra Demux/Selector in Simulink between inner_loop and this block.
%  Aileron is modelled here too now (1st-order lag + saturation), since it
%  is part of the same actuator_cmd vector and was previously handled
%  nowhere in the actuator-dynamics stage.
%
%  HARDWARE-READY BY DESIGN:
%    No persistent/global state and no Simulink-specific constructs. All
%    state is explicit in (act_state) and out (act_state_next); the only
%    external input is dt (seconds) and the parameter struct p. Same
%    signature a PX4 module would use per control-loop tick:
%    state_next = f(state, cmd, dt, params).
%
%    INTERNAL SUB-STEPPING: forward-Euler integration of the tilt 2nd-order
%    dynamics requires dt < p.dt_actuator_max (~0.1/tilt_omega_n) for
%    numerical stability. If the caller's dt exceeds this, this function
%    automatically sub-steps internally at p.dt_actuator_max so the OUTER
%    control loop rate is decoupled from the actuator model's numerical
%    stability requirement -- call this once per controller tick
%    regardless of dt; it self-subdivides. Port the same sub-stepping
%    logic to firmware if the flight computer's actuator-update rate is
%    slower than this bound.
%
%  ACTUATOR STATE LAYOUT (act_state, struct):
%    act_state.Omega(4)      rad/s   current motor speed (1st-order lag state)
%    act_state.beta(4)       rad     current tilt angle   (2nd-order lag state 1)
%    act_state.beta_dot(4)   rad/s   current tilt rate    (2nd-order lag state 2)
%    act_state.delta_ail     rad     current aileron deflection (1st-order lag)
%
%  INPUTS:
%    actuator_cmd(9x1)  [Omega_FL; Omega_FR; Omega_RL; Omega_RR;
%                         beta_FL;  beta_FR;  beta_RL;  beta_RR;
%                         delta_ail]   commanded values from dyulon_inner_loop,
%                         PRE-actuator-dynamics (this function's whole job
%                         is to turn these into what the hardware actually
%                         does a moment later)
%    dt                 s    CALLER's control step (any value -- this
%                              function sub-steps internally as needed)
%    p                       parameter struct from dyulon_init.m
%
%  OUTPUTS:
%    act_state_next            updated actuator state for next call
%    Omega_actual(4x1)  rad/s  actual (lagged, saturated) motor speed
%    beta_actual(4x1)   rad    actual (lagged, rate-limited, saturated) tilt
%    delta_ail_actual   rad    actual (lagged, saturated) aileron deflection
%    All three "actual" outputs feed dyulon_forces_moments as the 9x1
%    actuator_vec: [Omega_actual; beta_actual; delta_ail_actual].

%% --- Unpack the flat command vector ---
Omega_cmd = actuator_cmd(1:4);
beta_cmd  = actuator_cmd(5:8);
delta_ail_cmd = actuator_cmd(9);

%% --- Sub-stepping setup ---
n_sub  = max(1, ceil(dt / p.dt_actuator_max));
dt_sub = dt / n_sub;

Omega_i     = act_state.Omega;
beta_i      = act_state.beta;
betadot_i   = act_state.beta_dot;
delta_ail_i = act_state.delta_ail;

% Per-motor saturation (FIXED: was shared front/rear pair values, now
% genuinely per-motor to match p.beta_motor_min/max used by the controller).
Omega_cmd_sat = min(max(Omega_cmd, p.Omega_min(:)),      p.Omega_max(:));
beta_cmd_sat  = min(max(beta_cmd,  p.beta_motor_min(:)), p.beta_motor_max(:));
ail_cmd_sat   = min(max(delta_ail_cmd, p.aileron_min),   p.aileron_max);

for sub = 1:n_sub
    %% --- Motor speed: 1st-order lag, discretised, per-motor saturation ---
    % Continuous: Omega_dot = omega_c * (Omega_cmd - Omega)
    Omega_i = Omega_i + dt_sub * p.motor_bandwidth * (Omega_cmd_sat - Omega_i);
    Omega_i = min(max(Omega_i, p.Omega_min(:)), p.Omega_max(:));

    %% --- Tilt actuator: 2nd-order lag + hard rate limit, discretised ---
    % Continuous state-space (per motor), states [beta; beta_dot]:
    %   beta_dot_dot = omega_n^2*(beta_cmd - beta) - 2*zeta*omega_n*beta_dot
    % This law only acts on the numeric error (beta_cmd - beta), so it is
    % convention-agnostic -- works identically whether beta=0 means
    % horizontal (old unified convention) or up/down (current per-motor
    % convention), as long as beta_cmd and beta_i are expressed in the
    % SAME convention as each other, which they are (both come from/feed
    % the same per-motor beta values used throughout the cascade).
    betadotdot_i = p.tilt_omega_n^2 * (beta_cmd_sat - beta_i) ...
                 - 2 * p.tilt_zeta * p.tilt_omega_n * betadot_i;

    betadot_i = betadot_i + dt_sub * betadotdot_i;
    betadot_i = min(max(betadot_i, -p.tilt_rate_lim), p.tilt_rate_lim);

    beta_i = beta_i + dt_sub * betadot_i;
    beta_i = min(max(beta_i, p.beta_motor_min(:)), p.beta_motor_max(:));

    %% --- Aileron: 1st-order lag, discretised, saturation ---
    delta_ail_i = delta_ail_i + dt_sub * p.aileron_bandwidth * (ail_cmd_sat - delta_ail_i);
    delta_ail_i = min(max(delta_ail_i, p.aileron_min), p.aileron_max);
end

%% --- Pack outputs ---
act_state_next.Omega     = Omega_i;
act_state_next.beta      = beta_i;
act_state_next.beta_dot  = betadot_i;
act_state_next.delta_ail = delta_ail_i;

Omega_actual     = Omega_i;
beta_actual      = beta_i;
delta_ail_actual = delta_ail_i;

end

== matlab function Full_Model/Aircraft Dynamics/MATLAB Function1 ==
  data: uvw input; V_air output; alpha output; beta output
function [V_air, alpha, beta] = uvw_to_aero(uvw)
%#codegen
u = uvw(1); v = uvw(2); w = uvw(3);
V_air = sqrt(u^2 + v^2 + w^2);
V_air = max(V_air, 0.1);
alpha = atan2(w, u);
beta  = asin(v / V_air);
